simulink model "Random_Ball"  (R2016a)
settings: Solver=FixedStepDiscrete  StartTime=0.0  StopTime=inf  FixedStep=0.1  RelTol=1e-3
settings Model: Creator=DELL  LastModifiedBy=DELL
settings SolverCC: AutoInsertRateTranBlk=on
settings DataIOCC: LimitDataPoints=on
settings DebuggingCC: AllowSymbolicDim=off
settings ConfigComp: CovModelRefEnable=Off  CovSFcnEnable=off

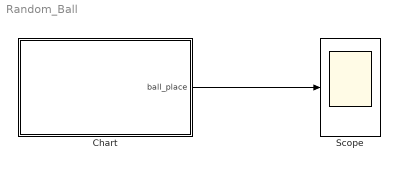
== system Random_Ball ==
  Chart : Stateflow chart  TreatAsAtomicUnit=on
  Scope : Scope
  wires:
  Chart/1(ball_place) -> Scope/1

== stateflow chart Random_Ball/Chart ==
  state Boundary_1
    entry: ball_place=1;
    ball=randi(400);
  state Boundary_2
    entry: ball_place=2;
    ball=randi(400);
  state Boundary_4
    entry: ball_place=4;
    ball=randi(300);
  state Boundary_3
    entry: ball_place=3;
    ball=randi(400);
  (default) -> Boundary_1
  Boundary_1 -> (junction 7) [order 1] : [ball<100 || (ball>100 && ball<200)]
  Boundary_1 -> (junction 8) [order 2] : [ball>300]
  (junction 7) -> Boundary_2 : [ball<100 || (ball>100 && ball<200)]
  (junction 8) -> Boundary_4 : [ball>300]
  (junction 22) -> Boundary_1 [order 1] : [ball<=100]
  Boundary_2 -> Boundary_1 [order 3] : [ball<100]
  Boundary_1 -> Boundary_3 [order 3] : [ball>200 && ball<=300]
  Boundary_3 -> Boundary_1 [order 3] : [ball<=100]
  Boundary_3 -> Boundary_4 [order 4] : [ball>200 && ball<=300]
  Boundary_2 -> (junction 22) [order 2] : [ball>300]
  Boundary_4 -> (junction 22) [order 2] : [ball<=100]
  (junction 22) -> Boundary_4 [order 2] : [ball>300]
  (junction 9) -> Boundary_4 [order 3] : [ball>300]
  (junction 10) -> Boundary_2 [order 2] : [ball>100 && ball<=200]
  Boundary_4 -> (junction 9) [order 1] : [ball>100]
  Boundary_2 -> Boundary_3 [order 4] : [ball>100 && ball<=200]
  Boundary_2 -> (junction 10) [order 1] : [ball>200 && ball<=300]
  Boundary_3 -> (junction 10) [order 2] : [ball>100 && ball<=200]
  Boundary_3 -> (junction 9) [order 1] : [ball>300]
  (junction 10) -> Boundary_3 [order 1] : [ball>200 && ball<=300]
  (junction 9) -> Boundary_3 [order 1] : [ball>200 && ball<=300]
  (junction 9) -> (junction 10) [order 2] : [ball>100 && ball<=200]
  data: ball_place output; ball local
